simulink model "servo_simulink"  (R2021b)
settings: Solver=VariableStepAuto  StartTime=0  StopTime=20  RelTol=1e-3
values from neighbouring files (symbols this model uses):
  A = [0, 0, 0, 1, 0, 0 ... (first row only)    [basic_data.m]    (also in basic_data.mat = [0 0 0 0 -22.4688936865 5 0 0 0 6.5 19.3959496459 -3.6 ... (; lqr.mat = [0 0 0 0 -22.4688936865 5 0 0 0 6.5 19.3959496459 -3.6 ... ()
  B = [0, 0 ... (first row only)    [basic_data.m]    (also in basic_data.mat = [0  0; 0  0; 0  0; 27  11.2; 6.06660129535  -1.63757677119; ; lqr.mat = [0  0; 0  0; 0  0; 27  11.2; 6.06660129535  -1.63757677119; )
  C = [1, 0, 0, 0, 0, 0 ... (first row only)    [basic_data.m]    (also in basic_data.mat = [1 0 0 0 1 0 0 0 1 0 0 0 ... (18 elements, 3x6)]; lqr.mat = [1 0 0 0 1 0 0 0 1 0 0 0 ... (18 elements, 3x6)])
  K = real(inv(R)*B'*P)    [ARE.m]    (also in LQR.m = inv(R)*B'*P; Pole_Placement_function.m = h/Wc*S; decoupled.m = F*C_star_star; lqr.mat = [-254.853126299  165.420589601  161.115517614  -14.472900470)
  x_0 = [0.2, -0.1, 0.15, -1, 0.8, 0]'    [basic_data.m]    (also in basic_data.mat = [0.2 -0.1 0.15 -1 0.8 0]; lqr.mat = [0.2 -0.1 0.15 -1 0.8 0])
  y_sp = -0.1*C*inv(A)*B*[-0.5+(a-b)/20;0.1+(b-c)/(a+d+10)]    [servo.m]
settings Model: Creator=asus  LastModifiedBy=asus
settings GRTTargetCC: RTWCAPISignals=on  RTWCAPIParams=on

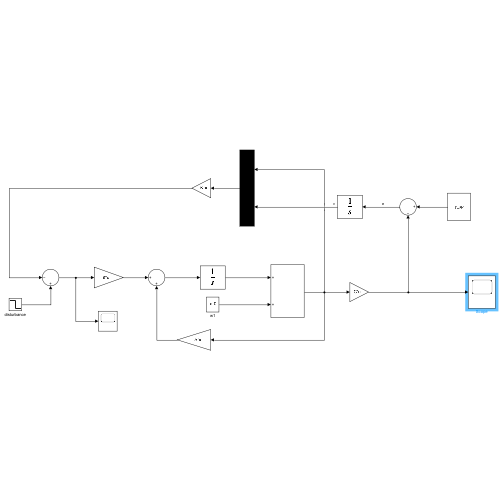
[thumbnail: Simulink's stored preview of the top-level diagram]
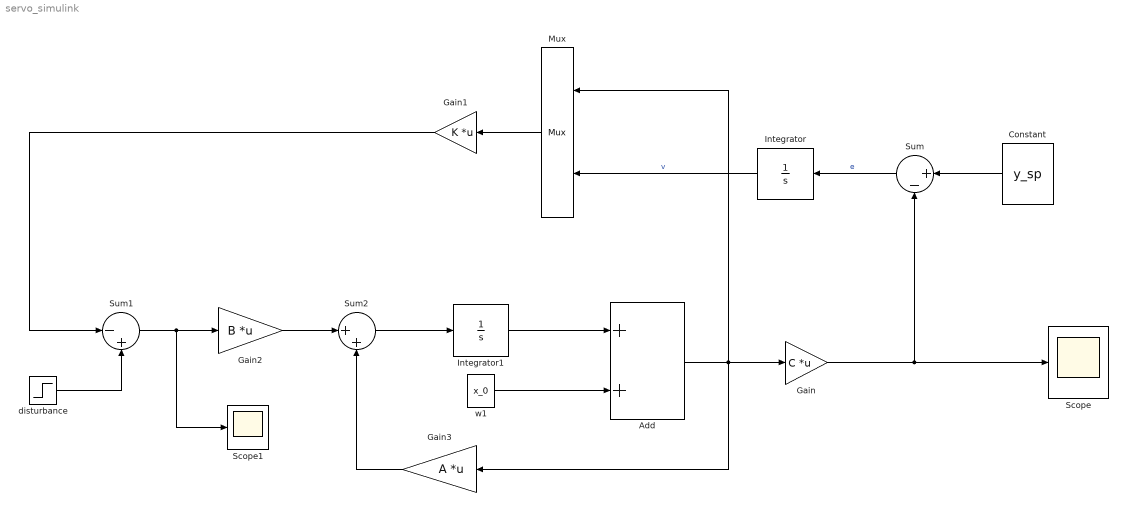
== system servo_simulink ==
  Add : Sum
  Constant : Constant  Value=y_sp
  Gain : Gain  Gain=C  Multiplication=Matrix(K*u)
  Gain1 : Gain  Gain=K  Multiplication=Matrix(K*u)
  Gain2 : Gain  Gain=B  Multiplication=Matrix(K*u)
  Gain3 : Gain  Gain=A  Multiplication=Matrix(K*u)
  Integrator : Integrator
  Integrator1 : Integrator
  Mux : Mux  Inputs=2
  Scope : Scope
  Scope1 : Scope
  Sum : Sum  Inputs=|+-
  Sum1 : Sum  Inputs=|-+
  Sum2 : Sum  Inputs=|++
  disturbance : Step  Time=10  Before=[0;0]  After=[-1;1]  SampleTime=0
  w1 : Constant  Value=x_0  VectorParams1D=off
  wires:
  Gain/1 -> Sum/2, Scope/1
  Constant/1 -> Sum/1
  Sum/1 -> Integrator/1  "e"
  Mux/1 -> Gain1/1
  Gain1/1 -> Sum1/1
  Gain2/1 -> Sum2/1
  Gain3/1 -> Sum2/2
  Sum2/1 -> Integrator1/1
  Integrator1/1 -> Add/1
  w1/1 -> Add/2
  disturbance/1 -> Sum1/2
  Sum1/1 -> Scope1/1, Gain2/1
  Integrator/1 -> Mux/2  "v"
  Add/1 -> Mux/1, Gain/1, Gain3/1
